simulink model "Convert_Celsius_Fahrenheit"  (R2021a)
settings: Solver=VariableStepAuto  StartTime=0.0  StopTime=10.0  RelTol=1e-3
settings Model: Creator=my computer  LastModifiedBy=my computer

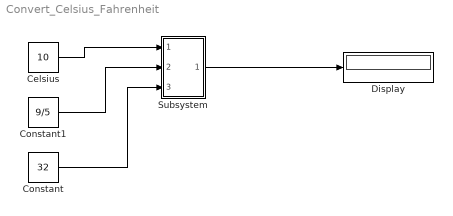
== system Convert_Celsius_Fahrenheit ==
  Celsius : Constant  Value=10
  Constant : Constant  Value=32
  Constant1 : Constant  Value=9/5
  Display : Display
  Subsystem : Subsystem
  wires:
  Celsius/1 -> Subsystem/1(Celsius)
  Constant1/1 -> Subsystem/2(In2)
  Constant/1 -> Subsystem/3(In3)
  Subsystem/1(Fahrenheit) -> Display/1

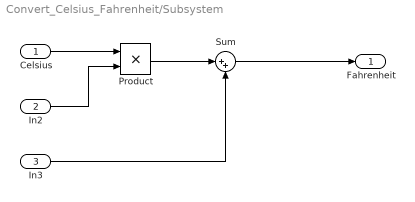
== system Convert_Celsius_Fahrenheit/Subsystem ==
  Celsius : Inport
  In2 : Inport  Port=2
  In3 : Inport  Port=3
  Product : Product
  Sum : Sum  Inputs=|++
  Fahrenheit : Outport
  wires:
  Celsius/1 -> Product/1
  Sum/1 -> Fahrenheit/1
  Product/1 -> Sum/1
  In3/1 -> Sum/2
  In2/1 -> Product/2
